simulink subsystem "DoublePulseFor6PulseRectifier"  (R2024a)
settings: Solver=VariableStepAuto  StartTime=0.0  StopTime=10.0  RelTol=1e-3
settings Model: Creator=Admin  LastModifiedBy=Admin

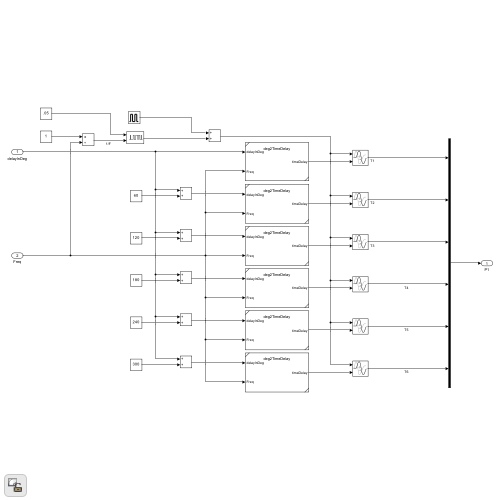
[thumbnail: Simulink's stored preview of the top-level diagram]
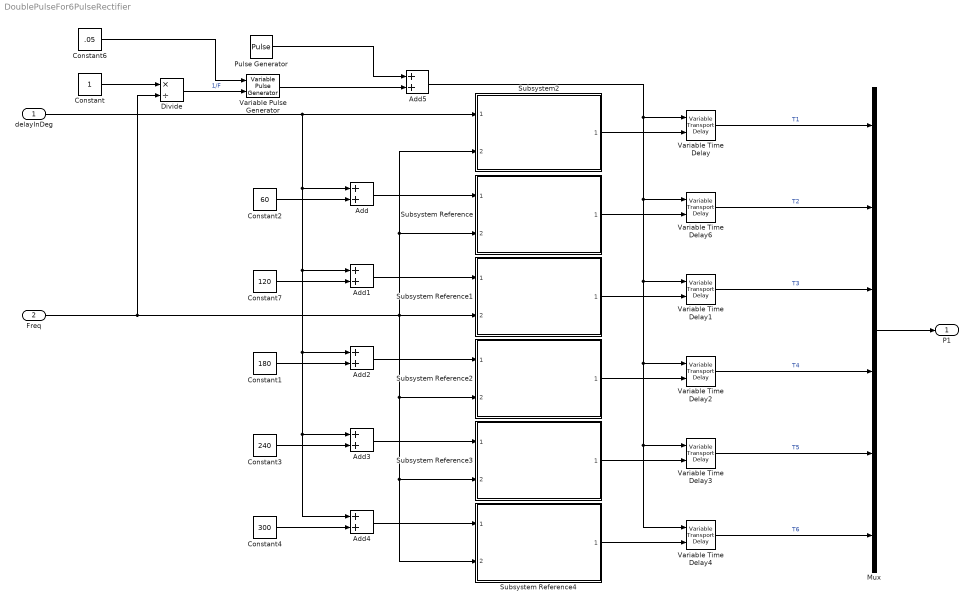
== system DoublePulseFor6PulseRectifier ==
  delayInDeg : Inport
  Freq : Inport  Port=2
  Add{,1..5} (6 alike) : Sum
  Constant : Constant
  Constant1 : Constant  Value=180
  Constant2 : Constant  Value=60
  Constant3 : Constant  Value=240
  Constant4 : Constant  Value=300
  Constant6 : Constant  Value=.05
  Constant7 : Constant  Value=120
  Divide : Product  Inputs=*/
  Mux : Mux  Inputs=6
  Pulse Generator : DiscretePulseGenerator  PulseType=Time based  Period=1/50  PulseWidth=5  PhaseDelay=(60/360)*(1/50)
  Subsystem Reference{,1..4} (5 alike) : Subsystem  ReferencedSubsystem=deg2TimeDelay
  Subsystem2 : Subsystem  ReferencedSubsystem=deg2TimeDelay
  Variable Time Delay{,1..4,6} (6 alike) : VariableTransportDelay  MaximumDelay=10  MaximumPoints=20000
  Variable Pulse Generator : VariablePulseGenerator  SampleTime=0.1
  P1 : Outport
  wires:
  Variable Time Delay3/1 -> Mux/5  "T5"
  Add5/1 -> Variable Time Delay/1, Variable Time Delay6/1, Variable Time Delay1/1, Variable Time Delay2/1, Variable Time Delay3/1, Variable Time Delay4/1
  Freq/1 -> Divide/2, Subsystem Reference1/2, Subsystem Reference2/2, Subsystem Reference3/2, Subsystem Reference4/2, Subsystem Reference/2, Subsystem2/2
  Variable Time Delay6/1 -> Mux/2  "T2"
  Variable Time Delay2/1 -> Mux/4  "T4"
  Variable Time Delay/1 -> Mux/1  "T1"
  Variable Time Delay4/1 -> Mux/6  "T6"
  Subsystem2/1 -> Variable Time Delay/2
  Variable Time Delay1/1 -> Mux/3  "T3"
  Subsystem Reference2/1 -> Variable Time Delay2/2
  Constant2/1 -> Add/2
  Constant1/1 -> Add2/2
  Subsystem Reference1/1 -> Variable Time Delay1/2
  Subsystem Reference4/1 -> Variable Time Delay4/2
  Constant4/1 -> Add4/2
  Subsystem Reference3/1 -> Variable Time Delay3/2
  delayInDeg/1 -> Subsystem2/1, Add/1, Add1/1, Add2/1, Add3/1, Add4/1
  Subsystem Reference/1 -> Variable Time Delay6/2
  Constant3/1 -> Add3/2
  Mux/1 -> P1/1
  Divide/1 -> Variable Pulse Generator/2  "1/F"
  Constant/1 -> Divide/1
  Constant6/1 -> Variable Pulse Generator/1
  Constant7/1 -> Add1/2
  Add1/1 -> Subsystem Reference1/1
  Add/1 -> Subsystem Reference/1
  Add2/1 -> Subsystem Reference2/1
  Add3/1 -> Subsystem Reference3/1
  Add4/1 -> Subsystem Reference4/1
  Variable Pulse Generator/1 -> Add5/2
  Pulse Generator/1 -> Add5/1
